simulink model "Final_Tune_of_Bandwidth_PI_Result"  (R2022b)
settings: Solver=FixedStepDiscrete  StartTime=0.0  StopTime=Inf  FixedStep=100e-6  RelTol=1e-3  EnableMultiTasking=on
undefined symbols (not defined in the file): C28x, CPU1, CPU2, CurrentBypassValue, DiscIntNeverNeededParam, Down, GPTRIP1SEL, TZ1, Up
libraries: c2802xlib x20, simulink x16, dspstat3 x10, dspsigops x6, c2837xDlib x5, PID_Lib x5, c280xlib x3, c2000lib x1
(part 1 of 3)
settings Model: ExtModeTrigDuration=8  Creator=user  LastModifiedBy=user
settings SolverCC: AutoInsertRateTranBlk=on
settings OptimizationCC: DefaultParameterBehavior=Inlined  DefaultUnderspecifiedDataType=single  EnhancedBackFolding=on  PassReuseOutputArgsAs=Individual arguments  MaxStackSize=1024  OptimizeBlockOrder=speed  DifferentSizesBufferReuse=on  OptimizationCustomize=off  DenormalBehavior=FlushToZero  EfficientTunableParamExpr=on
settings DebuggingCC: ParameterTunabilityLossMsg=error
settings HardwareCC: ProdBitPerChar=16  ProdBitPerInt=16  ProdBitPerPointer=32  ProdBitPerSizeT=32  ProdBitPerPtrDiffT=32  ProdLargestAtomicInteger=Integer  ProdLargestAtomicFloat=None  ProdWordSize=16  ProdLongLongMode=on  ProdHWDeviceType=Texas Instruments->C2000
settings ModelReferenceCC: ModelReferenceNumInstancesAllowed=Single
settings SFSimCC: MATLABDynamicMemAlloc=off
settings RTWCC: Description=Embedded Coder  SystemTargetFile=ert.tlc  HardwareBoard=TI Delfino F28379D LaunchPad  TLCOptions=-aInlineSetEventsForThisBaseRateFcn=TLC_FALSE -aSuppressMultiTaskScheduler=TLC_FALSE -aRateBasedStepFcn=1  TemplateMakefile=ert_default_tmf  GenerateReport=on  Toolchain=Texas Instruments Code Composer Studio (C2000)  LaunchReport=on
settings CodeAppCC: ForceParamTrailComments=on  IgnoreCustomStorageClasses=off  OperatorAnnotations=on  SimulinkDataObjDesc=on  SFDataObjDesc=on  InsertBlockDesc=on
settings ERTTargetCC: CodeReplacementLibrary=TI C28x  ExtModeTransport=4  ExtModeStaticAlloc=on  ExtModeStaticAllocSize=10000  ExtModeMexFile=ext_xcp  ExtModeIntrfLevel=Level2 - Open  InlinedParameterPlacement=NonHierarchical

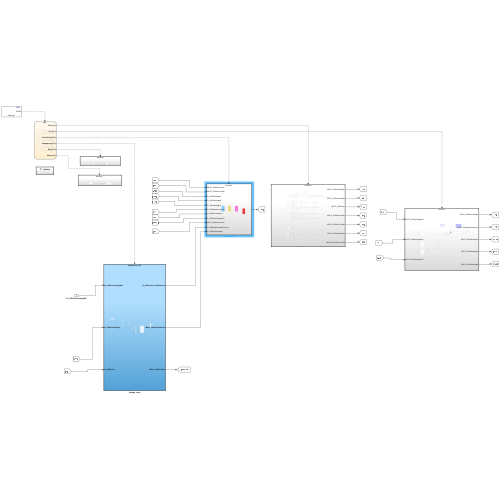
[thumbnail: Simulink's stored preview of the top-level diagram]
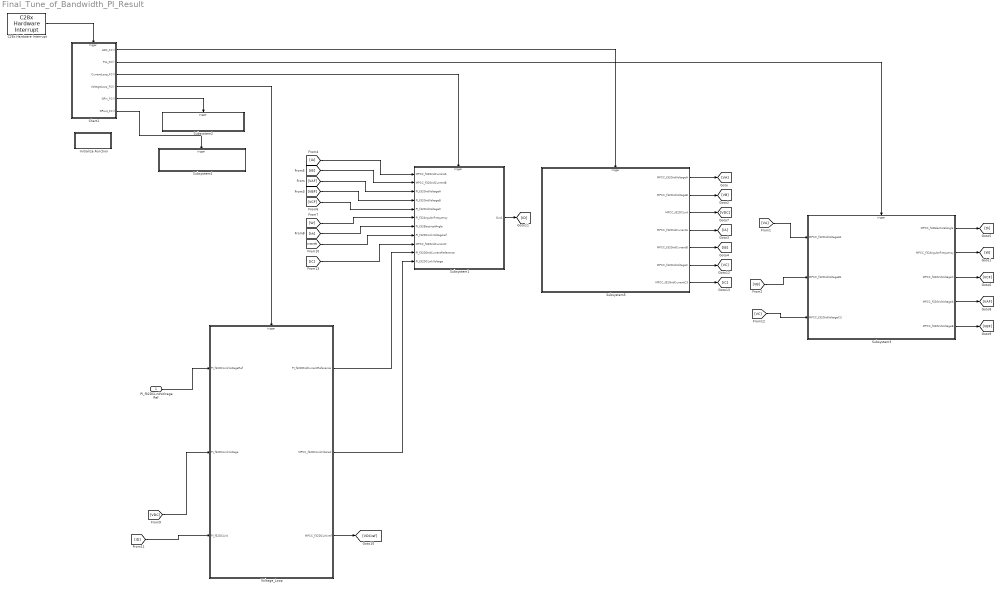
== system Final_Tune_of_Bandwidth_PI_Result ==
  PI_f32DCLinkVoltageRef : Inport
  C28x Hardware Interrupt : c2000lib/Scheduling/C28x Hardware Interrupt  irqnumbers=[1]  pienumbers=[1]  irqpriorities=[1]  irqpreempts=[1]  showinput=off  dspchiptype=C280X
  Chart1 : Stateflow chart  TreatAsAtomicUnit=on
  Initialize Function : Subsystem  TreatAsAtomicUnit=on
  Subsystem1 : Subsystem
  Subsystem2 : Subsystem
  Subsystem3 : Subsystem
  Subsystem4 : Subsystem
  Subsystem5 : Subsystem
  Voltage_Loop : Subsystem
  wires:
  Chart1/5(GPin_FC()) -> Subsystem2/Trigger
  Chart1/3(CurrentLoop_FC()) -> Subsystem1/Trigger
  Chart1/4(VoltageLoop_FC()) -> Voltage_Loop/Trigger
  C28x Hardware Interrupt/1 -> Chart1/Trigger
  Chart1/6(GPout_FC()) -> Subsystem4/Trigger
  Chart1/2(PLL_FC()) -> Subsystem3/Trigger
  Chart1/1(ADC_FC()) -> Subsystem5/Trigger
  Subsystem5/1(MPCC_f32GridVoltageA) -> [VA]
  Subsystem5/2(MPCC_f32GridVoltageB) -> [VB]
  [IA] -> Subsystem1/1(MPCC_f32GridCurrentA)
  [IB] -> Subsystem1/2(MPCC_f32GridCurrentB)
  [W] -> Subsystem1/6(PI_f32AngularFrequency)
  [th] -> Subsystem1/7(PI_f32ElectricalAngle)
  Subsystem5/3(MPCC_f32DCLink) -> [VDC]
  Voltage_Loop/2(MPCC_f32DCLinkFiltered) -> Subsystem1/11(PI_f32DCLinkVoltage)
  [VA] -> Subsystem3/1(MPCC_f32GridVoltageA2)
  [VAF] -> Subsystem1/3(PI_f32GridVoltageA)
  [VCF] -> Subsystem1/5(PI_f32GridVoltageC)
  [VBF] -> Subsystem1/4(PI_f32GridVoltageB)
  Subsystem5/4(MPCC_f32GridCurrentA) -> [IA]
  Subsystem5/5(MPCC_f32GridCurrentB) -> [IB]
  Voltage_Loop/3(MPCC_f32DCLinkref) -> [VDCref]
  [VDCref] -> Subsystem1/8(PI_f32DCLinkVoltageref)
  [VDC] -> Voltage_Loop/2(PI_f32DCLinkVoltage)
  PI_f32DCLinkVoltageRef/1 -> Voltage_Loop/1(PI_f32DCLinkVoltageRef)
  Voltage_Loop/1(PI_f32DGridCurrentReference) -> Subsystem1/10(PI_f32DGridCurrentReference)
  Subsystem1/1(Out1) -> [ID]
  [ID] -> Voltage_Loop/3(PI_f32DCLink)
  [VB] -> Subsystem3/2(MPCC_f32GridVoltageB1)
  Subsystem5/6(MPCC_f32GridVoltageC) -> [VC]
  Subsystem5/7(MPCC_f32GridCurrentC3) -> [IC]
  [VC] -> Subsystem3/3(MPCC_f32GridVoltageC3)
  [IC] -> Subsystem1/9(MPCC_f32GridCurrentC)
  Subsystem3/1(MPCC_f32ElectricalAngle) -> [th]
  Subsystem3/2(MPCC_f32AngularFrequency) -> [W]
  Subsystem3/3(MPCC_f32GridVoltageC) -> [VCF]
  Subsystem3/4(MPCC_f32GridVoltageA) -> [VAF]
  Subsystem3/5(MPCC_f32GridVoltageB) -> [VBF]

== system Final_Tune_of_Bandwidth_PI_Result/Initialize Function ==
  Constant : Constant  Value=boolean(0)
  Digital Output : c2837xDlib/Digital Output  GPIO_Number=GPIO8~GPIO15  GPIO_Bit0=off  GPIO_BIT0_Toggle=off  GPIO_Bit1=off  GPIO_BIT1_Toggle=off  GPIO_Bit2=off  GPIO_BIT2_Toggle=off  GPIO_Bit3=on  GPIO_BIT3_Toggle=off  GPIO_Bit4=off  GPIO_BIT4_Toggle=off  GPIO_Bit5=off  GPIO_BIT5_Toggle=off  GPIO_Bit6=off  GPIO_BIT6_Toggle=off  GPIO_Bit7=off  GPIO_BIT7_Toggle=off
  Event Listener : EventListener  DisableCoverage=on  EventName=reset
  wires:
  Constant/1 -> Digital Output/1

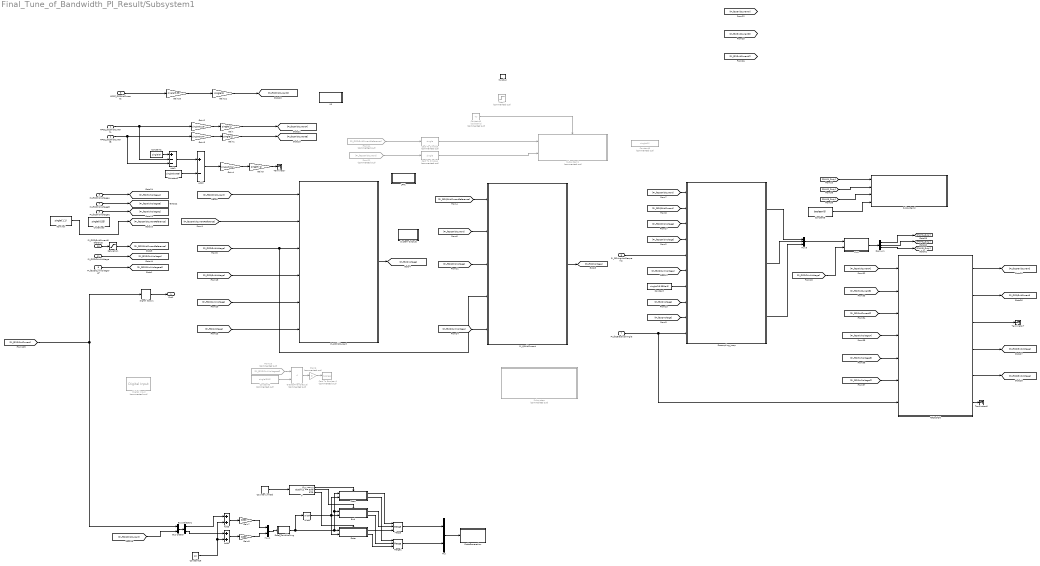
== system Final_Tune_of_Bandwidth_PI_Result/Subsystem1 ==
  MPCC_f32GridCurrentA : Inport
  MPCC_f32GridCurrentB : Inport  Port=2
  PI_f32GridVoltageA : Inport  Port=3
  PI_f32GridVoltageB : Inport  Port=4
  PI_f32GridVoltageC : Inport  Port=5
  PI_f32AngularFrequency : Inport  Port=6
  PI_f32ElectricalAngle : Inport  Port=7
  PI_f32DCLinkVoltageref : Inport  Port=8
  MPCC_f32GridCurrentC : Inport  Port=9
  PI_f32DGridCurrentReference : Inport  Port=10
  PI_f32DCLinkVoltage : Inport  Port=11
  function : TriggerPort  TriggerType=function-call  VariantControl=(inherit)
  ABCtoDQO : Subsystem
  Add1 : Sum  Inputs=+--
  Add2 : Sum  Inputs=+-
  Add3 : Sum
  Add4 : Sum
  Bus Creator : BusCreator  Inputs=2
  Bus Selector1 : BusSelector  OutputSignals=signal1,signal2
  Cast To Boolean1 : DataTypeConversion  Commented=on  OutDataTypeStr=boolean  SaturateOnIntegerOverflow=off  RndMeth=Floor
  Cast To Single3 : DataTypeConversion  Commented=on  OutDataTypeStr=single  SaturateOnIntegerOverflow=off  RndMeth=Floor
  Cast To Single4 : DataTypeConversion  Commented=on  OutDataTypeStr=single  SaturateOnIntegerOverflow=off  RndMeth=Floor
  CodeGeneration : Subsystem  TreatAsAtomicUnit=on
  Constant : Constant  Value=single(18.355e-3)
  Constant1 : Constant  Value=single(0)
  Constant16 : Constant  Value=10  OutDataTypeStr=single
  Constant2 : Constant  Value=single(0.005)
  Constant3 : Constant  Commented=on  Value=boolean(1)
  Constant5 : Constant  Value=boolean(0)
  Constant6 : Constant  Commented=on  Value=single(300)
  Constant9 : Constant  Commented=on  Value=single(0)
  Counter Limited : simulink/Sources/Counter Limited  uplimit=599  tsamp=-1
  Data : Subsystem  TreatAsAtomicUnit=on
  Data_Conditioning : Subsystem
  Decoupling_Loop : Subsystem
  Demux1 : Demux  Outputs=3
  Digital Input : c280xlib/Digital Input  Commented=on  GPIO_Number=GPIO32~GPIO34  GPIO_Bit0=on  GPIO_Bit1=off  GPIO_Bit2=off  GPIO_Bit3=off  GPIO_Bit4=off  GPIO_Bit5=off  GPIO_Bit6=off  GPIO_Bit7=off  sampleTime=-1  dataType=boolean  GPIO_Bit0_Qualification=Sync to SYSCLKOUT  GPIO_Bit1_Qualification=Sync to SYSCLKOUT  GPIO_Bit2_Qualification=Sync to SYSCLKOUT  GPIO_Bit3_Qualification=Sync to SYSCLKOUT  GPIO_Bit4_Qualification=Sync to SYSCLKOUT  GPIO_Bit5_Qualification=Sync to SYSCLKOUT  GPIO_Bit6_Qualification=Sync to SYSCLKOUT  GPIO_Bit7_Qualification=Sync to SYSCLKOUT  Qualification_Period=-1
  End : Subsystem  TreatAsAtomicUnit=on
  From14 : From  Commented=on  GotoTag=PI_f32DGridCurrentReference
  From16 : From  Commented=on  GotoTag=PI_f32DCLinkVoltageref
  From21 : From  Commented=on  GotoTag=PI_f32DGridCurrent
  Gain : Gain  Gain=single(1)
  Gain1 : Gain  Gain=single(1)
  Gain2 : Gain  Gain=single(6.25)
  Gain20 : Gain  Gain=single(5.85)
  Gain21 : Gain  Gain=single(1)
  Gain3 : Gain  Gain=single(5.94)
  Gain4 : Gain  Gain=single(5.94)
  Gain5 : Gain  Gain=single(-1)
  Gain6 : Gain  Commented=on  Gain=0
  Gain7 : Gain  Gain=1000  OutDataTypeStr=single
  Gain8 : Gain  Gain=1000  OutDataTypeStr=single
  GreaterThanOrEqual : RelationalOperator  Commented=on  Operator=<  OutDataTypeStr=boolean  RndMeth=Simplest  InputSameDT=off
  IIR : Subsystem
  If : If  IfExpression=u1 == 0  ElseIfExpressions=u1 == 599
  LPF1 : Subsystem
  Merge : Merge  Inputs=3
  Merge1 : Merge  Inputs=3
  Mux : Mux  Inputs=2
  Mux1 : Mux  Inputs=2
  Mux5 : Mux  Inputs=3
  Nominal : Constant  Value=single(1.1)  VectorParams1D=off  SampleTime=-1
  PI_DGridCurrent : Subsystem
  PI_QGridCurrent : Subsystem
  SVM : Subsystem
  Saturation : Saturate  UpperLimit=7  LowerLimit=-7
  Signal Copy1 : SignalConversion  OverrideOpt=off
  Start : Subsystem  TreatAsAtomicUnit=on
  Step1 : Step  Commented=on  Time=70
  Subsystem : Subsystem  Commented=on
  Subsystem1 : Subsystem  Commented=on
  Subsystem2 : Subsystem
  System Outputs : Subsystem  mask(System Outputs){ShowInLibBrowser=0}
      mask prompts: ShowInLibBrowser "Simulink:masks:CustCodeMaskParam1_MP"
      settings: CopyFcn=cccopyfcn(gcb)  OpenFcn=ccopenfcn('System Outputs Function')
      mask Help: eval('feval(''rtwprivate'',''rtwhelpview'',''rtw_sys_outputs_block'')');
      mask Display: disp('System\nOutputs');
  Terminator : Terminator
  Terminator6 : Terminator
  Terminator7 : Terminator
  Underload : Constant  Value=single(0.55)  VectorParams1D=off  SampleTime=-1
  Width : Width  OutDataTypeMode=All ports same datatype  DataType=uint16
  Out1 : Outport
  wires:
  Add1/1 -> Add2/1
  Gain2/1 -> Gain/1  "Iau"
  Constant2/1 -> Add2/2
  Add2/1 -> Gain4/1
  Gain4/1 -> Gain5/1  "Icu"
  MPCC_f32GridCurrentA/1 -> Gain2/1, Add1/2
  Gain3/1 -> Gain1/1  "Ibu"
  MPCC_f32GridCurrentB/1 -> Add1/3, Gain3/1
  Constant1/1 -> Add1/1
  [PI_f32QGridVoltage] -> Decoupling_Loop/4(PI_f32QGridVoltage)
  [PI_f32QVoltage] -> Decoupling_Loop/9(PI_f32QVoltage)
  [PI_f32QGridCurrentReference] -> PI_QGridCurrent/1(PI_f32QGridCurrentReference)
  [PI_f32QGridCurrent] -> Decoupling_Loop/2(PI_f32QGridCurrent)
  [PI_f32QGridCurrent] -> PI_QGridCurrent/2(PI_f32QGridCurrent)
  [PI_f32DGridVoltage] -> Decoupling_Loop/3(PI_f32DGridVoltage)
  Constant/1 -> Decoupling_Loop/7(PI_f32LGrid)
  [PI_f32DCLinkVoltage] -> Decoupling_Loop/6(PI_f32DCLinkVoltage)
  [PI_f32DGridCurrent] -> Decoupling_Loop/1(PI_f32DGridCurrent)
  PI_QGridCurrent/1(PI_f32QVoltage) -> [PI_f32QVoltage]
  PI_f32AngularFrequency/1 -> Decoupling_Loop/5(PI_f32AngularFrequency)
  PI_DGridCurrent/1(PI_f32DVoltage) -> [PI_f32DVoltage]
  [PI_f32DVoltage] -> Decoupling_Loop/8(PI_f32DVoltage)
  [PI_f32GridCurrentA] -> ABCtoDQO/1(PI_f32GridCurrentA)
  ABCtoDQO/6(PI_f32OGridVoltage) -> Terminator6/1
  [PI_f32GridVoltageB] -> ABCtoDQO/5(PI_f32GridVoltageB)
  ABCtoDQO/1(PI_f32DGridCurrent) -> [PI_f32DGridCurrent]
  [PI_f32GridVoltageC] -> ABCtoDQO/6(PI_f32GridVoltageC)
  ABCtoDQO/5(PI_f32QGridVoltage) -> [PI_f32QGridVoltage]
  [PI_f32GridCurrentB] -> ABCtoDQO/2(PI_f32GridCurrentB)
  [PI_f32GridCurrentC] -> ABCtoDQO/3(PI_f32GridCurrentC)
  ABCtoDQO/3(PI_f32OGridCurrent) -> Terminator7/1
  ABCtoDQO/2(PI_f32QGridCurrent) -> [PI_f32QGridCurrent]
  ABCtoDQO/4(PI_f32DGridVoltage) -> [PI_f32DGridVoltage]
  PI_f32GridVoltageC/1 -> [PI_f32GridVoltageC]
  PI_f32GridVoltageB/1 -> [PI_f32GridVoltageB]
  PI_f32GridVoltageA/1 -> [PI_f32GridVoltageA]
  Gain/1 -> [PI_f32GridCurrentA]
  Gain1/1 -> [PI_f32GridCurrentB]
  Gain5/1 -> Terminator/1
  PI_f32ElectricalAngle/1 -> ABCtoDQO/7(PI_f32ElectricalAngle), Decoupling_Loop/10(PI_f32ElectricalAngle)
  [PI_f32DGridCurrent] -> PI_DGridCurrent/1(PI_f32DGridCurrent)
  PI_f32DCLinkVoltage/1 -> [PI_f32DCLinkVoltage]
  [PI_f32DGridVoltage] -> PI_QGridCurrent/4(PI_f32DGridVoltage), PI_DGridCurrent/3(PI_f32DGridVoltage)
  [PI_f32QGridVoltage] -> PI_QGridCurrent/3(PI_f32QGridVoltage)
  [PI_f32QGridVoltage] -> PI_DGridCurrent/4(PI_f32QGridVoltage)
  [PI_f32GridVoltageA] -> ABCtoDQO/4(PI_f32GridVoltageA)
  [PI_f32DCLinkVoltage] -> PI_DGridCurrent/5(PI_f32DCLinkVoltage)
  [PI_f32QVoltage] -> PI_DGridCurrent/6(PI_f32QVoltage)
  [PI_f32DCLinkVoltage] -> PI_QGridCurrent/5(PI_f32DCLinkVoltage)
  PI_f32DCLinkVoltageref/1 -> [PI_f32DCLinkVoltageref]
  Saturation/1 -> [PI_f32DGridCurrentReference]
  PI_f32DGridCurrentReference/1 -> Saturation/1
  From16/1 -> GreaterThanOrEqual/1
  Constant6/1 -> GreaterThanOrEqual/2
  GreaterThanOrEqual/1 -> Gain6/1
  Cast To Single4/1 -> Subsystem1/2(In2)
  Cast To Single3/1 -> Subsystem1/1(In1)
  From21/1 -> Cast To Single4/1
  From14/1 -> Cast To Single3/1
  Signal Copy1/1 -> Out1/1
  Constant3/1 -> Subsystem1/Enable
  MPCC_f32GridCurrentC/1 -> Gain20/1
  Gain21/1 -> [PI_f32GridCurrentC]  "Iau"
  Gain20/1 -> Gain21/1  "Iau"
  Gain6/1 -> Cast To Boolean1/1
  Demux1/2 -> [PWM2_Duty]
  SVM/1(Dabc) -> Demux1/1
  Demux1/3 -> [PWM3_Duty]
  Demux1/1 -> [PWM1_Duty]
  Decoupling_Loop/2(PI_f32MBVoltageRef) -> Mux5/2
  Decoupling_Loop/1(PI_f32MAVoltageRef) -> Mux5/1
  Decoupling_Loop/3(PI_f32MCVoltageRef) -> Mux5/3
  Mux5/1 -> SVM/1(Vabc)
  [PI_f32DCLinkVoltage] -> SVM/2(Vdc)
  [PWM1_Duty] -> Subsystem2/1(PWM1)
  [PWM2_Duty] -> Subsystem2/2(PWM2)
  [PWM3_Duty] -> Subsystem2/3(PWM3)
  Constant5/1 -> Subsystem2/4(Trip)
  [PI_f32DGridCurrent] -> Signal Copy1/1, Bus Creator/1
  [PI_f32DGridCurrentReference] -> PI_DGridCurrent/2(PI_f32DGridCurrentReference)
  Start/2(Iteration) -> Merge1/1
  Gain8/1 -> Mux1/2
  Data/2(Iteration) -> Merge1/3
  Bus Selector1/1 -> Add3/1  "<signal1>"
  Counter Limited/1 -> If/1
  If/3 -> Data/Action
  End/1(Data_out) -> Merge/2
  If/1 -> Start/Action
  If/2 -> End/Action
  Width/1 -> Data/2(Data_width), Start/2(Data_width), End/2(Data_width)
  Data_Conditioning/1(Out1) -> Width/1, Start/1(Data), End/1(Data), Data/1(Data)
  Merge/1 -> Mux/1  "SCI_Tx_Data"
  End/2(Iteration) -> Merge1/2
  Merge1/1 -> Mux/2  "SCI_Tx_Iteration"
  Start/1(Data_out) -> Merge/1
  Add3/1 -> Gain7/1
  Bus Creator/1 -> Bus Selector1/1
  Gain7/1 -> Mux1/1
  Mux/1 -> CodeGeneration/1(Input)
  Constant16/1 -> Add3/2, Add4/2
  Bus Selector1/2 -> Add4/1  "<signal2>"
  Data/1(Data_out) -> Merge/3
  Mux1/1 -> Data_Conditioning/1(In1)
  [PI_f32QGridCurrent] -> Bus Creator/2
  Add4/1 -> Gain8/1
  Nominal/1 -> [PI_f32QGridCurrentReference]

== system Final_Tune_of_Bandwidth_PI_Result/Subsystem2 ==
  function : TriggerPort  TriggerType=function-call  VariantControl=(inherit)
  Constant : Constant  Value=boolean(1)
  Digital Output : c2837xDlib/Digital Output  GPIO_Number=GPIO8~GPIO15  GPIO_Bit0=off  GPIO_BIT0_Toggle=off  GPIO_Bit1=off  GPIO_BIT1_Toggle=off  GPIO_Bit2=off  GPIO_BIT2_Toggle=off  GPIO_Bit3=off  GPIO_BIT3_Toggle=off  GPIO_Bit4=off  GPIO_BIT4_Toggle=off  GPIO_Bit5=off  GPIO_BIT5_Toggle=off  GPIO_Bit6=on  GPIO_BIT6_Toggle=off  GPIO_Bit7=off  GPIO_BIT7_Toggle=off
  wires:
  Constant/1 -> Digital Output/1

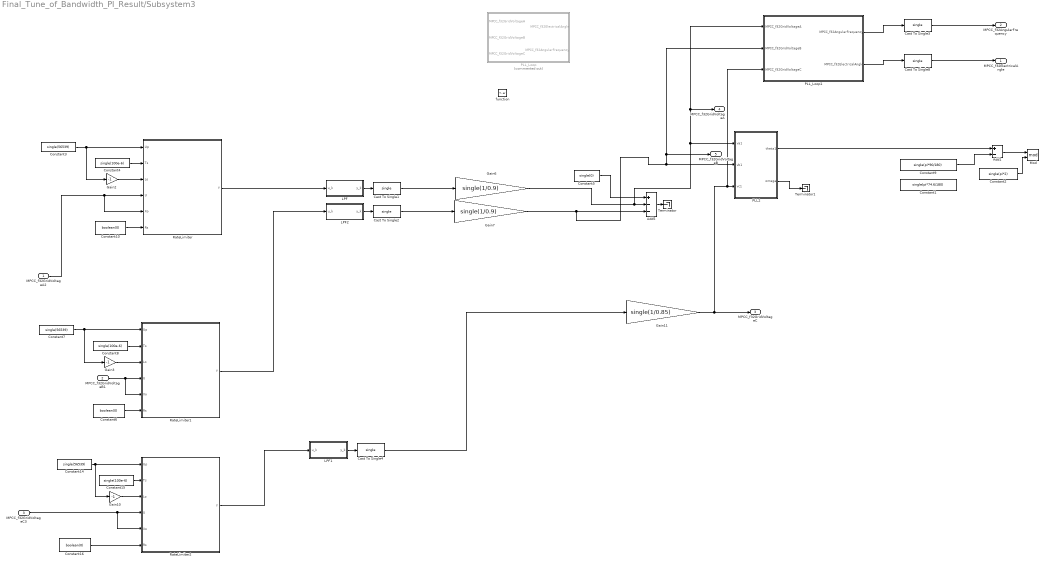
== system Final_Tune_of_Bandwidth_PI_Result/Subsystem3 ==
  MPCC_f32GridVoltageA2 : Inport
  MPCC_f32GridVoltageB1 : Inport  Port=2
  MPCC_f32GridVoltageC3 : Inport  Port=3
  function : TriggerPort  TriggerType=function-call  VariantControl=(inherit)
  Add1 : Sum  Inputs=+-
  Add5 : Sum  Inputs=+--
  Cast To Single{1..4,8} (5 alike) : DataTypeConversion  OutDataTypeStr=single  SaturateOnIntegerOverflow=off  RndMeth=Floor
  Constant1 : Constant  Value=single(pi*74.6/180)
  Constant10 : Constant  Value=boolean(0)
  Constant14 : Constant  Value=single(56539)
  Constant15 : Constant  Value=single(100e-6)
  Constant16 : Constant  Value=boolean(0)
  Constant2 : Constant  Value=single(pi*2)
  Constant3 : Constant  Value=single(56539)
  Constant4 : Constant  Value=single(100e-6)
  Constant5 : Constant  Value=single(0)
  Constant6 : Constant  Value=boolean(0)
  Constant7 : Constant  Value=single(56539)
  Constant8 : Constant  Value=single(100e-6)
  Constant9 : Constant  Value=single(pi*90/180)
  Gain10 : Gain  Gain=-1
  Gain11 : Gain  Gain=single(1/0.85)
  Gain2 : Gain  Gain=-1
  Gain3 : Gain  Gain=-1
  Gain6 : Gain  Gain=single(1/0.9)
  Gain7 : Gain  Gain=single(1/0.9)
  LPF : Subsystem
  LPF1 : Subsystem
  LPF2 : Subsystem
  Mod : Math  Operator=mod
  PLL2 : Subsystem
  PLL_Loop : Subsystem  Commented=on  TreatAsAtomicUnit=on
  PLL_Loop1 : Subsystem
  RateLimiter : Subsystem
  RateLimiter1 : Subsystem
  RateLimiter2 : Subsystem
  Terminator : Terminator
  Terminator1 : Terminator
  MPCC_f32ElectricalAngle : Outport
  MPCC_f32AngularFrequency : Outport  Port=2
  MPCC_f32GridVoltageC : Outport  Port=3
  MPCC_f32GridVoltageA : Outport  Port=4
  MPCC_f32GridVoltageB : Outport  Port=5
  wires:
  Cast To Single1/1 -> Gain6/1
  Constant5/1 -> Add5/1
  Cast To Single2/1 -> Gain7/1
  Constant2/1 -> Mod/2
  PLL2/1(theta1) -> Add1/1
  Add1/1 -> Mod/1
  LPF/1(y_k) -> Cast To Single1/1
  LPF2/1(y_k) -> Cast To Single2/1
  Gain6/1 -> PLL_Loop1/1(MPCC_f32GridVoltageA), MPCC_f32GridVoltageA/1, PLL2/1(va1), Add5/2
  Gain7/1 -> MPCC_f32GridVoltageB/1, PLL_Loop1/2(MPCC_f32GridVoltageB), PLL2/2(vb1), Add5/3
  Gain2/1 -> RateLimiter/3(Lo)
  Constant10/1 -> RateLimiter/6(Rs)
  Constant3/1 -> Gain2/1, RateLimiter/1(Up)
  Constant4/1 -> RateLimiter/2(Ts)
  MPCC_f32GridVoltageA2/1 -> RateLimiter/5(Xo), RateLimiter/4(U)
  RateLimiter/1(Y) -> LPF/1(u_k)
  Constant7/1 -> Gain3/1, RateLimiter1/1(Up)
  Constant6/1 -> RateLimiter1/6(Rs)
  Constant8/1 -> RateLimiter1/2(Ts)
  Gain3/1 -> RateLimiter1/3(Lo)
  MPCC_f32GridVoltageB1/1 -> RateLimiter1/5(Xo), RateLimiter1/4(U)
  RateLimiter1/1(Y) -> LPF2/1(u_k)
  MPCC_f32GridVoltageC3/1 -> RateLimiter2/5(Xo), RateLimiter2/4(U)
  Cast To Single4/1 -> Gain11/1
  LPF1/1(y_k) -> Cast To Single4/1
  Constant14/1 -> Gain10/1, RateLimiter2/1(Up)
  Constant15/1 -> RateLimiter2/2(Ts)
  Constant16/1 -> RateLimiter2/6(Rs)
  Gain10/1 -> RateLimiter2/3(Lo)
  RateLimiter2/1(Y) -> LPF1/1(u_k)
  Add5/1 -> Terminator/1
  Gain11/1 -> PLL2/3(vc1), PLL_Loop1/3(MPCC_f32GridVoltageC), MPCC_f32GridVoltageC/1
  Constant9/1 -> Add1/2
  Cast To Single8/1 -> MPCC_f32ElectricalAngle/1
  Cast To Single3/1 -> MPCC_f32AngularFrequency/1
  PLL_Loop1/2(MPCC_f32ElectricalAngle) -> Cast To Single8/1
  PLL_Loop1/1(MPCC_f32AngularFrequency) -> Cast To Single3/1
  PLL2/2(omega) -> Terminator1/1

== system Final_Tune_of_Bandwidth_PI_Result/Subsystem4 ==
  function : TriggerPort  TriggerType=function-call  VariantControl=(inherit)
  Constant : Constant  Value=boolean(0)
  Digital Output : c2837xDlib/Digital Output  GPIO_Number=GPIO8~GPIO15  GPIO_Bit0=off  GPIO_BIT0_Toggle=off  GPIO_Bit1=off  GPIO_BIT1_Toggle=off  GPIO_Bit2=off  GPIO_BIT2_Toggle=off  GPIO_Bit3=off  GPIO_BIT3_Toggle=off  GPIO_Bit4=off  GPIO_BIT4_Toggle=off  GPIO_Bit5=off  GPIO_BIT5_Toggle=off  GPIO_Bit6=on  GPIO_BIT6_Toggle=off  GPIO_Bit7=off  GPIO_BIT7_Toggle=off
  wires:
  Constant/1 -> Digital Output/1

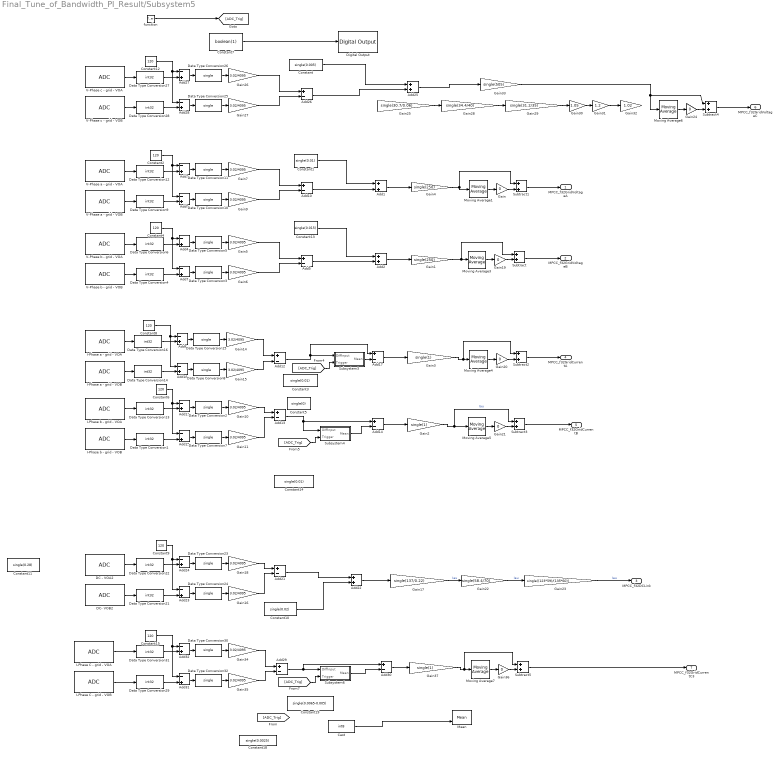
== system Final_Tune_of_Bandwidth_PI_Result/Subsystem5 ==
  function : TriggerPort  TriggerType=function-call  VariantControl=(inherit)  ShowOutputPort=on  OutputDataType=int8
  Add{1..2,22,25} (4 alike) : Sum  AccumDataTypeStr=single  OutDataTypeStr=single
  Add{5,10,12..14,17,21,26,29..30} (10 alike) : Sum  Inputs=+-  AccumDataTypeStr=single  OutDataTypeStr=single
  Add{3..4,6..7,9,11,15,18,23..24,27..28,31..32} (14 alike) : Sum  Inputs=-+  AccumDataTypeStr=single  OutDataTypeStr=single
  Cast : DataTypeConversion  OutDataTypeStr=int8  SaturateOnIntegerOverflow=off  RndMeth=Floor
  Constant : Constant  Value=single(0.005)
  Constant1 : Constant  Value=single(0.01)
  Constant10 : Constant  Value=single(0.02)
  Constant11 : Constant  Value=single(0.28)
  Constant{2,4,6,8..9,12,15} (7 alike) : Constant  Value=120  OutDataTypeStr=single
  Constant13 : Constant  Value=single(0.015)
  Constant14 : Constant  Value=single(0.01)
  Constant18 : Constant  Value=single(0.0025)
  Constant19 : Constant  Value=single(0.0065-0.005)
  Constant3 : Constant  Value=single(0.01)
  Constant5 : Constant  Value=single(0)
  Constant7 : Constant  Value=boolean(1)
  DC - VOA2 : c2802xlib/ADC  blkParamProc=C2000_Type4  ADCModule=C  samplingMode=Single sample mode  ADCResolution=12-bit (Single-ended input)  useSOC1=SOC0  useSOC2=SOC0_SOC1  SOCAcquisitionWindow=22  SOCTriggerSource=ePWM1_ADCSOCA  SOCInterruptTrigger=No ADCINT  Ts=-1  dType=uint16  postInterrupt=off  interruptSel=ADCINT1  ADCINTContinuous=on  endma=off  chdma=1  conv1=ADCINA0  conv2=ADCINA0 and ADCINB0  conv1_Type4=ADCIN5  conv2_Type4=ADCIN0 and ADCIN1
  DC- VOB2 : c2802xlib/ADC  blkParamProc=C2000_Type4  ADCModule=B  samplingMode=Single sample mode  ADCResolution=12-bit (Single-ended input)  useSOC1=SOC3  useSOC2=SOC0_SOC1  SOCAcquisitionWindow=22  SOCTriggerSource=ePWM1_ADCSOCA  SOCInterruptTrigger=No ADCINT  Ts=-1  dType=uint16  postInterrupt=off  interruptSel=ADCINT2  ADCINTContinuous=on  endma=off  chdma=1  conv1=ADCINA0  conv2=ADCINA0 and ADCINB0  conv1_Type4=ADCIN5  conv2_Type4=ADCIN2 and ADCIN3
  Data Type Conversion{1,4,6,9,12..14,16,21..22,27..29,31} (14 alike) : DataTypeConversion  OutDataTypeStr=int32  ConvertRealWorld=Stored Integer (SI)  SaturateOnIntegerOverflow=off  RndMeth=Floor
  Data Type Conversion{2..3,5,7..8,10..11,15,23..26,30,32} (14 alike) : DataTypeConversion  OutDataTypeStr=single  SaturateOnIntegerOverflow=off  RndMeth=Floor
  Digital Output : c2837xDlib/Digital Output  GPIO_Number=GPIO32~GPIO39  GPIO_Bit0=on  GPIO_BIT0_Toggle=on  GPIO_Bit1=off  GPIO_BIT1_Toggle=off  GPIO_Bit2=off  GPIO_BIT2_Toggle=off  GPIO_Bit3=off  GPIO_BIT3_Toggle=off  GPIO_Bit4=off  GPIO_BIT4_Toggle=off  GPIO_Bit5=off  GPIO_BIT5_Toggle=off  GPIO_Bit6=off  GPIO_BIT6_Toggle=off  GPIO_Bit7=off  GPIO_BIT7_Toggle=off
  Gain{,19..21,24,36} (6 alike) : Gain  Gain=0
  Gain1 : Gain  Gain=single(250)
  Gain{5..7,9..11,14..16,18,26..27,34..35} (14 alike) : Gain  Gain=3.02/4095  ParamDataTypeStr=single  OutDataTypeStr=single
  Gain17 : Gain  Gain=single(137/0.22)
  Gain2 : Gain  Gain=single(1)
  Gain22 : Gain  Gain=single(58.4/70)
  Gain23 : Gain  Gain=single((123*59)/(135*60))
  Gain25 : Gain  Gain=single(30.7/0.06)
  Gain28 : Gain  Gain=single(34.4/40)
  Gain29 : Gain  Gain=single(31.2/35)
  Gain3 : Gain  Gain=single(1)
  Gain30 : Gain  Gain=1.05
  Gain31 : Gain  Gain=1.2
  Gain32 : Gain  Gain=1.02
  Gain33 : Gain  Gain=single(505)
  Gain37 : Gain  Gain=single(1)
  Gain4 : Gain  Gain=single(250)
  I-Phase C - grid - VOA : c2802xlib/ADC  blkParamProc=C2000_Type4  ADCModule=A  samplingMode=Single sample mode  ADCResolution=12-bit (Single-ended input)  useSOC1=SOC15  useSOC2=SOC0_SOC1  SOCAcquisitionWindow=22  SOCTriggerSource=ePWM1_ADCSOCA  SOCInterruptTrigger=No ADCINT  Ts=-1  dType=uint16  postInterrupt=off  interruptSel=ADCINT1  ADCINTContinuous=on  endma=off  chdma=1  conv1=ADCINA0  conv2=ADCINA0 and ADCINB0  conv1_Type4=ADCIN15  conv2_Type4=ADCIN0 and ADCIN1
  I-Phase C - grid - VOB : c2802xlib/ADC  blkParamProc=C2000_Type4  ADCModule=A  samplingMode=Single sample mode  ADCResolution=12-bit (Single-ended input)  useSOC1=SOC10  useSOC2=SOC0_SOC1  SOCAcquisitionWindow=22  SOCTriggerSource=ePWM1_ADCSOCA  SOCInterruptTrigger=No ADCINT  Ts=-1  dType=uint16  postInterrupt=off  interruptSel=ADCINT2  ADCINTContinuous=on  endma=off  chdma=1  conv1=ADCINA0  conv2=ADCINA0 and ADCINB0  conv1_Type4=ADCIN14  conv2_Type4=ADCIN2 and ADCIN3
  I-Phase a - grid - VOA : c2802xlib/ADC  blkParamProc=C2000_Type4  ADCModule=A  samplingMode=Single sample mode  ADCResolution=12-bit (Single-ended input)  useSOC1=SOC0  useSOC2=SOC0_SOC1  SOCAcquisitionWindow=22  SOCTriggerSource=ePWM1_ADCSOCA  SOCInterruptTrigger=No ADCINT  Ts=-1  dType=uint16  postInterrupt=on  interruptSel=ADCINT1  ADCINTContinuous=on  endma=off  chdma=1  conv1=ADCINA0  conv2=ADCINA0 and ADCINB0  conv1_Type4=ADCIN4  conv2_Type4=ADCIN0 and ADCIN1
  I-Phase a - grid - VOB : c2802xlib/ADC  blkParamProc=C2000_Type4  ADCModule=B  samplingMode=Single sample mode  ADCResolution=12-bit (Single-ended input)  useSOC1=SOC1  useSOC2=SOC0_SOC1  SOCAcquisitionWindow=22  SOCTriggerSource=ePWM1_ADCSOCA  SOCInterruptTrigger=No ADCINT  Ts=-1  dType=uint16  postInterrupt=off  interruptSel=ADCINT2  ADCINTContinuous=on  endma=off  chdma=1  conv1=ADCINA0  conv2=ADCINA0 and ADCINB0  conv1_Type4=ADCIN4  conv2_Type4=ADCIN2 and ADCIN3
  I-Phase b - grid - VOA : c2802xlib/ADC  blkParamProc=C2000_Type4  ADCModule=C  samplingMode=Single sample mode  ADCResolution=12-bit (Single-ended input)  useSOC1=SOC12  useSOC2=SOC0_SOC1  SOCAcquisitionWindow=22  SOCTriggerSource=ePWM1_ADCSOCA  SOCInterruptTrigger=No ADCINT  Ts=-1  dType=uint16  postInterrupt=off  interruptSel=ADCINT1  ADCINTContinuous=on  endma=off  chdma=1  conv1=ADCINA0  conv2=ADCINA0 and ADCINB0  conv1_Type4=ADCIN4  conv2_Type4=ADCIN0 and ADCIN1
  I-Phase b - grid - VOB : c2802xlib/ADC  blkParamProc=C2000_Type4  ADCModule=A  samplingMode=Single sample mode  ADCResolution=12-bit (Single-ended input)  useSOC1=SOC3  useSOC2=SOC0_SOC1  SOCAcquisitionWindow=22  SOCTriggerSource=ePWM1_ADCSOCA  SOCInterruptTrigger=No ADCINT  Ts=-1  dType=uint16  postInterrupt=off  interruptSel=ADCINT2  ADCINTContinuous=on  endma=off  chdma=1  conv1=ADCINA0  conv2=ADCINA0 and ADCINB0  conv1_Type4=ADCIN5  conv2_Type4=ADCIN2 and ADCIN3
  Mean : dspstat3/Mean  run=on  InputProcessing=Columns as channels (frame based)  reset_popup=Rising edge  directionMode=Each column  dimension=1  roiEnable=off  roiType=Rectangles  roiPortion=Entire ROI  roiOutput=Individual statistics for each ROI  roiFlag=off  roundingMode=Floor  overflowMode=off  outputDataTypeStr=Inherit: Same as accumulator  outputMin=[]  outputMax=[]  outputLastDataTypeStr=Inherit: Same as accumulator
  Moving Average{1,3..7} (6 alike) : dspstat3/Moving Average  Method=Exponential weighting  ForgettingFactorPort=off  SpecifyWindowLength=on  WindowLength=4  OverlapLength=3  AllowArbitraryInputLength=off  ForgettingFactor=0.99  SimulateUsing=Code generation
  Subsystem3 : Subsystem
  Subsystem4 : Subsystem
  Subsystem6 : Subsystem
  Subtract{,1..5} (6 alike) : Sum
  V-Phase a - grid - VOA : c2802xlib/ADC  blkParamProc=C2000_Type4  ADCModule=C  samplingMode=Single sample mode  ADCResolution=12-bit (Single-ended input)  useSOC1=SOC4  useSOC2=SOC0_SOC1  SOCAcquisitionWindow=22  SOCTriggerSource=ePWM1_ADCSOCA  SOCInterruptTrigger=No ADCINT  Ts=-1  dType=uint16  postInterrupt=off  interruptSel=ADCINT1  ADCINTContinuous=on  endma=off  chdma=1  conv1=ADCINA0  conv2=ADCINA0 and ADCINB0  conv1_Type4=ADCIN3  conv2_Type4=ADCIN0 and ADCIN1
  V-Phase a - grid - VOB : c2802xlib/ADC  blkParamProc=C2000_Type4  ADCModule=B  samplingMode=Single sample mode  ADCResolution=12-bit (Single-ended input)  useSOC1=SOC5  useSOC2=SOC0_SOC1  SOCAcquisitionWindow=22  SOCTriggerSource=ePWM1_ADCSOCA  SOCInterruptTrigger=No ADCINT  Ts=-1  dType=uint16  postInterrupt=off  interruptSel=ADCINT2  ADCINTContinuous=on  endma=off  chdma=1  conv1=ADCINA0  conv2=ADCINA0 and ADCINB0  conv1_Type4=ADCIN3  conv2_Type4=ADCIN2 and ADCIN3
  V-Phase b - grid - VOA : c2802xlib/ADC  blkParamProc=C2000_Type4  ADCModule=A  samplingMode=Single sample mode  ADCResolution=12-bit (Single-ended input)  useSOC1=SOC6  useSOC2=SOC0_SOC1  SOCAcquisitionWindow=22  SOCTriggerSource=ePWM1_ADCSOCA  SOCInterruptTrigger=No ADCINT  Ts=-1  dType=uint16  postInterrupt=off  interruptSel=ADCINT1  ADCINTContinuous=on  endma=off  chdma=1  conv1=ADCINA0  conv2=ADCINA0 and ADCINB0  conv1_Type4=ADCIN3  conv2_Type4=ADCIN0 and ADCIN1
  V-Phase b - grid - VOB : c2802xlib/ADC  blkParamProc=C2000_Type4  ADCModule=C  samplingMode=Single sample mode  ADCResolution=12-bit (Single-ended input)  useSOC1=SOC7  useSOC2=SOC0_SOC1  SOCAcquisitionWindow=22  SOCTriggerSource=ePWM1_ADCSOCA  SOCInterruptTrigger=No ADCINT  Ts=-1  dType=uint16  postInterrupt=off  interruptSel=ADCINT2  ADCINTContinuous=on  endma=off  chdma=1  conv1=ADCINA0  conv2=ADCINA0 and ADCINB0  conv1_Type4=ADCIN2  conv2_Type4=ADCIN2 and ADCIN3
  V-Phase c - grid - VOA : c2802xlib/ADC  blkParamProc=C2000_Type4  ADCModule=B  samplingMode=Single sample mode  ADCResolution=12-bit (Single-ended input)  useSOC1=SOC0  useSOC2=SOC0_SOC1  SOCAcquisitionWindow=22  SOCTriggerSource=ePWM1_ADCSOCA  SOCInterruptTrigger=No ADCINT  Ts=-1  dType=uint16  postInterrupt=off  interruptSel=ADCINT1  ADCINTContinuous=on  endma=off  chdma=1  conv1=ADCINA0  conv2=ADCINA0 and ADCINB0  conv1_Type4=ADCIN2  conv2_Type4=ADCIN0 and ADCIN1
  V-Phase c - grid - VOB : c2802xlib/ADC  blkParamProc=C2000_Type4  ADCModule=A  samplingMode=Single sample mode  ADCResolution=12-bit (Single-ended input)  useSOC1=SOC1  useSOC2=SOC0_SOC1  SOCAcquisitionWindow=22  SOCTriggerSource=ePWM1_ADCSOCA  SOCInterruptTrigger=No ADCINT  Ts=-1  dType=uint16  postInterrupt=off  interruptSel=ADCINT2  ADCINTContinuous=on  endma=off  chdma=1  conv1=ADCINA0  conv2=ADCINA0 and ADCINB0  conv1_Type4=ADCIN2  conv2_Type4=ADCIN2 and ADCIN3
  MPCC_f32GridVoltageA : Outport
  MPCC_f32GridVoltageB : Outport  Port=2
  MPCC_f32DCLink : Outport  Port=3
  MPCC_f32GridCurrentA : Outport  Port=4
  MPCC_f32GridCurrentB : Outport  Port=5
  MPCC_f32GridVoltageC : Outport  Port=6
  MPCC_f32GridCurrentC3 : Outport  Port=7
  wires:
  Gain5/1 -> Add5/1
  Data Type Conversion5/1 -> Gain5/1
  Gain1/1 -> Subtract/1, Moving Average3/1
  Add9/1 -> Data Type Conversion10/1
  V-Phase a - grid - VOB/1 -> Data Type Conversion9/1
  Data Type Conversion9/1 -> Add9/2
  Gain7/1 -> Add10/1
  Data Type Conversion10/1 -> Gain9/1
  Data Type Conversion12/1 -> Add3/2
  Add7/1 -> Data Type Conversion3/1
  Data Type Conversion4/1 -> Add7/2
  Data Type Conversion6/1 -> Add4/2
  Gain9/1 -> Add10/2
  V-Phase b - grid - VOB/1 -> Data Type Conversion4/1
  V-Phase b - grid - VOA/1 -> Data Type Conversion6/1
  Add4/1 -> Data Type Conversion5/1
  Add3/1 -> Data Type Conversion11/1
  Data Type Conversion3/1 -> Gain6/1
  Gain6/1 -> Add5/2
  Constant4/1 -> Add7/1, Add4/1
  V-Phase a - grid - VOA/1 -> Data Type Conversion12/1
  Constant2/1 -> Add9/1, Add3/1
  Data Type Conversion11/1 -> Gain7/1
  Add1/1 -> Gain4/1
  Add2/1 -> Gain1/1
  I-Phase b - grid - VOA/1 -> Data Type Conversion13/1
  Data Type Conversion15/1 -> Gain14/1
  Data Type Conversion8/1 -> Gain15/1
  Data Type Conversion14/1 -> Add18/2
  Gain15/1 -> Add12/2
  Data Type Conversion13/1 -> Add11/2
  Data Type Conversion16/1 -> Add6/2
  Gain14/1 -> Add12/1
  Add6/1 -> Data Type Conversion15/1
  Gain10/1 -> Add13/1
  Add18/1 -> Data Type Conversion8/1
  I-Phase a - grid - VOA/1 -> Data Type Conversion16/1
  Gain2/1 -> Subtract3/1, Moving Average5/1  "Iau"
  Data Type Conversion2/1 -> Gain10/1
  Constant6/1 -> Add15/1, Add11/1
  I-Phase b - grid - VOB/1 -> Data Type Conversion1/1
  Data Type Conversion1/1 -> Add15/2
  Gain11/1 -> Add13/2
  Add17/1 -> Gain3/1
  Add11/1 -> Data Type Conversion2/1
  Constant8/1 -> Add18/1, Add6/1
  I-Phase a - grid - VOB/1 -> Data Type Conversion14/1
  Data Type Conversion7/1 -> Gain11/1
  Add15/1 -> Data Type Conversion7/1
  Subtract/1 -> MPCC_f32GridVoltageB/1
  Moving Average3/1 -> Gain19/1
  Moving Average1/1 -> Gain/1
  Gain4/1 -> Subtract1/1, Moving Average1/1
  Subtract1/1 -> MPCC_f32GridVoltageA/1
  Moving Average4/1 -> Gain20/1
  Gain3/1 -> Subtract2/1, Moving Average4/1
  Moving Average5/1 -> Gain21/1
  Data Type Conversion22/1 -> Add24/2
  DC- VOB2/1 -> Data Type Conversion21/1
  Data Type Conversion21/1 -> Add23/2
  Data Type Conversion23/1 -> Gain18/1
  DC - VOA2/1 -> Data Type Conversion22/1
  Add24/1 -> Data Type Conversion23/1
  Constant9/1 -> Add23/1, Add24/1
  Gain16/1 -> Add21/2
  Add23/1 -> Data Type Conversion24/1
  Data Type Conversion24/1 -> Gain16/1
  Gain18/1 -> Add21/1
  Gain/1 -> Subtract1/2
  Gain19/1 -> Subtract/2
  Gain20/1 -> Subtract2/2
  Gain21/1 -> Subtract3/2
  Gain17/1 -> Gain22/1  "Iau"
  Subtract2/1 -> MPCC_f32GridCurrentA/1
  Subtract3/1 -> MPCC_f32GridCurrentB/1
  Gain22/1 -> Gain23/1  "Iau"
  V-Phase c - grid - VOB/1 -> Data Type Conversion28/1
  Gain26/1 -> Add26/1
  Data Type Conversion25/1 -> Gain27/1
  V-Phase c - grid - VOA/1 -> Data Type Conversion27/1
  Subtract4/1 -> MPCC_f32GridVoltageC/1
  Data Type Conversion26/1 -> Gain26/1
  Data Type Conversion27/1 -> Add27/2
  Moving Average6/1 -> Gain24/1
  Data Type Conversion28/1 -> Add28/2
  Gain27/1 -> Add26/2
  Add28/1 -> Data Type Conversion25/1
  Constant12/1 -> Add28/1, Add27/1
  Add27/1 -> Data Type Conversion26/1
  Gain25/1 -> Gain28/1
  Gain24/1 -> Subtract4/2
  Gain28/1 -> Gain29/1
  Gain29/1 -> Gain30/1
  Gain30/1 -> Gain31/1
  Gain31/1 -> Gain32/1
  Gain33/1 -> Subtract4/1, Moving Average6/1
  Add31/1 -> Data Type Conversion32/1
  Data Type Conversion32/1 -> Gain35/1
  Data Type Conversion31/1 -> Add32/2
  Gain34/1 -> Add29/1
  Constant15/1 -> Add31/1, Add32/1
  Gain35/1 -> Add29/2
  Subtract5/1 -> MPCC_f32GridCurrentC3/1
  Gain36/1 -> Subtract5/2
  Data Type Conversion30/1 -> Gain34/1
  Data Type Conversion29/1 -> Add31/2
  I-Phase C - grid - VOB/1 -> Data Type Conversion29/1
  I-Phase C - grid - VOA/1 -> Data Type Conversion31/1
  Gain37/1 -> Subtract5/1, Moving Average7/1
  Add32/1 -> Data Type Conversion30/1
  Add30/1 -> Gain37/1
  Moving Average7/1 -> Gain36/1
  Add22/1 -> Gain17/1
  Constant7/1 -> Digital Output/1
  Add14/1 -> Gain2/1
  function/1 -> [ADC_Trig]
  Cast/1 -> Mean/2
  Add25/1 -> Gain33/1
  [ADC_Trig] -> Subsystem3/2(Trigger)
  Add12/1 -> Add17/1, Subsystem3/1(DiffInput)
  Subsystem3/1(Mean) -> Add17/2
  [ADC_Trig] -> Subsystem4/2(Trigger)
  Add13/1 -> Add14/1, Subsystem4/1(DiffInput)
  Subsystem4/1(Mean) -> Add14/2
  [ADC_Trig] -> Subsystem6/2(Trigger)
  Add29/1 -> Add30/1, Subsystem6/1(DiffInput)
  Subsystem6/1(Mean) -> Add30/2
  Constant/1 -> Add25/1
  Add26/1 -> Add25/2
  Constant1/1 -> Add1/1
  Add10/1 -> Add1/2
  Constant13/1 -> Add2/1
  Add5/1 -> Add2/2
  Gain23/1 -> MPCC_f32DCLink/1  "Iau"
  Add21/1 -> Add22/1
  Constant10/1 -> Add22/2

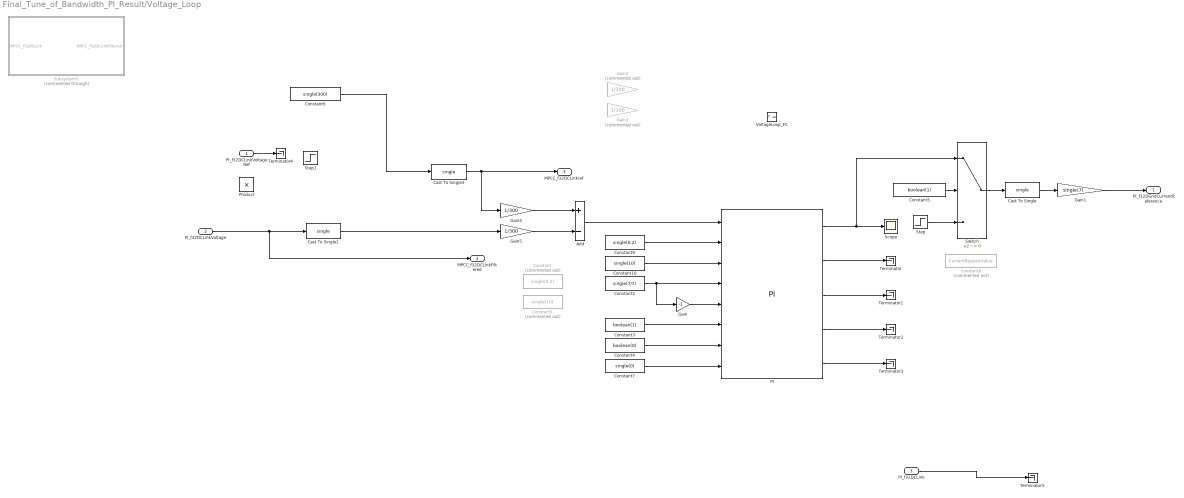
== system Final_Tune_of_Bandwidth_PI_Result/Voltage_Loop ==
  PI_f32DCLinkVoltageRef : Inport
  PI_f32DCLinkVoltage : Inport  Port=2
  PI_f32DCLink : Inport  Port=3
  VoltageLoop_FC : TriggerPort  TriggerType=function-call  VariantControl=(inherit)  SampleTime=-1
      settings: AttributesFormatString=|
      | %<StatesWhenEnabling>
      | %<SampleTime>
  Add : Sum  Inputs=+-
  Cast To Single : DataTypeConversion  OutDataTypeStr=single  SaturateOnIntegerOverflow=off  RndMeth=Floor
  Cast To Single1 : DataTypeConversion  OutDataTypeStr=single  SaturateOnIntegerOverflow=off  RndMeth=Floor
  Cast To Single3 : DataTypeConversion  OutDataTypeStr=single  SaturateOnIntegerOverflow=off  RndMeth=Floor
  Constant : Constant  Commented=on  Value=single(0.2)
  Constant1 : Constant  Commented=on  Value=single(10)
  Constant10 : Constant  Value=single(10)
  Constant2 : Constant  Value=single(7/7)
  Constant3 : Constant  Value=boolean(1)
  Constant4 : Constant  Value=boolean(0)
  Constant5 : Constant  Value=boolean(1)
  Constant6 : Constant  Value=single(300)
  Constant7 : Constant  Value=single(0)
  Constant8 : Constant  Commented=on  Value=CurrentBypassValue
  Constant9 : Constant  Value=single(0.2)
  Gain : Gain  Gain=-1
  Gain1 : Gain  Gain=single(7)
  Gain2 : Gain  Commented=on  Gain=1/100
  Gain3 : Gain  Commented=on  Gain=1/100
  Gain4 : Gain  Gain=1/300
  Gain5 : Gain  Gain=1/300
  PI : PID_Lib/PI  SystemSampleTime=-1  VariantActivationTime=update diagram  Latency=0  AutoFrameSizeCalculation=off
  Product : Product
  Scope : Scope
  Step : Step  Time=30  Before=-0.5  After=-1.5
  Step1 : Step  Time=50  Before=200  After=300
  Subsystem5 : Subsystem  Commented=through
  Switch : Switch  Criteria=u2 ~= 0  SaturateOnIntegerOverflow=off  InputSameDT=off
  Terminator{,1..5} (6 alike) : Terminator
  PI_f32DGridCurrentReference : Outport
  MPCC_f32DCLinkFiltered : Outport  Port=2
  MPCC_f32DCLinkref : Outport  Port=3
  wires:
  Add/1 -> PI/1
  Constant2/1 -> Gain/1, PI/4
  Gain/1 -> PI/5
  Constant3/1 -> PI/6
  Constant4/1 -> PI/7
  PI/2 -> Terminator/1
  PI/3 -> Terminator1/1
  PI/4 -> Terminator2/1
  PI/5 -> Terminator3/1
  Constant5/1 -> Switch/2
  PI/1 -> Switch/1, Scope/1
  Switch/1 -> Cast To Single/1
  Cast To Single1/1 -> Gain5/1
  Cast To Single/1 -> Gain1/1
  Cast To Single3/1 -> Gain4/1, MPCC_f32DCLinkref/1
  PI_f32DCLinkVoltage/1 -> Cast To Single1/1, MPCC_f32DCLinkFiltered/1
  Constant7/1 -> PI/8
  Step/1 -> Switch/3
  Gain1/1 -> PI_f32DGridCurrentReference/1
  PI_f32DCLinkVoltageRef/1 -> Terminator4/1
  PI_f32DCLink/1 -> Terminator5/1
  Constant9/1 -> PI/2
  Constant10/1 -> PI/3
  Gain4/1 -> Add/1
  Gain5/1 -> Add/2
  Constant6/1 -> Cast To Single3/1

== system Final_Tune_of_Bandwidth_PI_Result/Subsystem1/ABCtoDQO ==
  PI_f32GridCurrentA : Inport
  PI_f32GridCurrentB : Inport  Port=2
  PI_f32GridCurrentC : Inport  Port=3
  PI_f32GridVoltageA : Inport  Port=4
  PI_f32GridVoltageB : Inport  Port=5
  PI_f32GridVoltageC : Inport  Port=6
  PI_f32ElectricalAngle : Inport  Port=7
  ABCtoDQOCurrent : Subsystem  Commented=on
  ABCtoDQOVoltage : Subsystem  Commented=on
  Ground : Ground
  abc_dq : Subsystem
  abc_dq1 : Subsystem
  PI_f32DGridCurrent : Outport
  PI_f32QGridCurrent : Outport  Port=2
  PI_f32OGridCurrent : Outport  Port=3
  PI_f32DGridVoltage : Outport  Port=4
  PI_f32QGridVoltage : Outport  Port=5
  PI_f32OGridVoltage : Outport  Port=6
  wires:
  abc_dq/1(Id) -> PI_f32DGridCurrent/1
  abc_dq/2(Iq) -> PI_f32QGridCurrent/1
  PI_f32ElectricalAngle/1 -> [PI_f32ElectricalAngle]
  [PI_f32ElectricalAngle] -> abc_dq/1(theta)
  Ground/1 -> PI_f32OGridCurrent/1, PI_f32OGridVoltage/1
  abc_dq1/2(Iq) -> PI_f32QGridVoltage/1
  [PI_f32ElectricalAngle] -> abc_dq1/1(theta)
  abc_dq1/1(Id) -> PI_f32DGridVoltage/1
  PI_f32GridCurrentC/1 -> abc_dq/4(c)
  PI_f32GridCurrentB/1 -> abc_dq/3(b)
  PI_f32GridCurrentA/1 -> abc_dq/2(a)
  PI_f32GridVoltageA/1 -> abc_dq1/2(a)
  PI_f32GridVoltageB/1 -> abc_dq1/3(b)
  PI_f32GridVoltageC/1 -> abc_dq1/4(c)

== system Final_Tune_of_Bandwidth_PI_Result/Subsystem1/CodeGeneration ==
  Input : Inport
  Add : Sum  Inputs=+-  OutDataTypeStr=Inherit: Same as first input
  Demux2 : Demux  Outputs=2
  Index Vector : MultiPortSwitch  Inputs=1  SaturateOnIntegerOverflow=off  InputSameDT=off
  SCI Transmit : c280xlib/SCI Transmit  sciModule=A  dataHead=''  dataTail=''  blockingMode=on  outputStatus=off
  While Iterator : WhileIterator  MaxIters=-1  WhileBlockType=do-while  ShowIterationPort=on  OutputDataType=int16
  wires:
  While Iterator/1 -> Add/2, Index Vector/1
  Demux2/1 -> Index Vector/2
  Index Vector/1 -> SCI Transmit/1
  Add/1 -> While Iterator/1
  Demux2/2 -> Add/1
  Input/1 -> Demux2/1

== system Final_Tune_of_Bandwidth_PI_Result/Subsystem1/Data ==
  Data : Inport
  Data_width : Inport  Port=2
  Action Port : ActionPort  ActionPortLabel=else
  Mux : Mux  Inputs=2
  Start : Constant  Value=hex2dec('0000')  OutDataTypeStr=uint16
  Data_out : Outport  VectorParamsAs1DForOutWhenUnconnected=off
  Iteration : Outport  Port=2  VectorParamsAs1DForOutWhenUnconnected=off
  wires:
  Start/1 -> Mux/2
  Mux/1 -> Data_out/1
  Data/1 -> Mux/1
  Data_width/1 -> Iteration/1

== system Final_Tune_of_Bandwidth_PI_Result/Subsystem1/Data_Conditioning ==
  In1 : Inport
  Data Type Conversion3 : DataTypeConversion  OutDataTypeStr=uint16  ConvertRealWorld=Stored Integer (SI)  SaturateOnIntegerOverflow=off  RndMeth=Floor
  Out1 : Outport  VectorParamsAs1DForOutWhenUnconnected=off
  wires:
  Data Type Conversion3/1 -> Out1/1
  In1/1 -> Data Type Conversion3/1

== system Final_Tune_of_Bandwidth_PI_Result/Subsystem1/Decoupling_Loop ==
  PI_f32DGridCurrent : Inport
  PI_f32QGridCurrent : Inport  Port=2
  PI_f32DGridVoltage : Inport  Port=3
  PI_f32QGridVoltage : Inport  Port=4
  PI_f32AngularFrequency : Inport  Port=5
  PI_f32DCLinkVoltage : Inport  Port=6
  PI_f32LGrid : Inport  Port=7
  PI_f32DVoltage : Inport  Port=8
  PI_f32QVoltage : Inport  Port=9
  PI_f32ElectricalAngle : Inport  Port=10
  ABCtoDQOVoltage : Subsystem  Commented=on
  Cast To Single : DataTypeConversion  OutDataTypeStr=single  SaturateOnIntegerOverflow=off  RndMeth=Floor
  Cast To Single1 : DataTypeConversion  OutDataTypeStr=single  SaturateOnIntegerOverflow=off  RndMeth=Floor
  Cast To Single2 : DataTypeConversion  OutDataTypeStr=single  SaturateOnIntegerOverflow=off  RndMeth=Floor
  Constant : Constant  Value=single(0)
  Decoupling_Loop : Subsystem
  Saturation : Saturate  Commented=on  UpperLimit=single(2/sqrt(3))  LowerLimit=single(-2/sqrt(3))
  Saturation1 : Saturate  Commented=on  UpperLimit=single(2/sqrt(3))  LowerLimit=single(-2/sqrt(3))
  Scope : Scope
  Scope1 : Scope
  Terminator : Terminator
  dq_abc : Subsystem
  PI_f32MAVoltageRef : Outport
  PI_f32MBVoltageRef : Outport  Port=2
  PI_f32MCVoltageRef : Outport  Port=3
  wires:
  PI_f32DGridCurrent/1 -> Decoupling_Loop/1(PI_f32DGridCurrent)
  PI_f32QGridCurrent/1 -> Decoupling_Loop/2(PI_f32QGridCurrent)
  PI_f32DGridVoltage/1 -> Decoupling_Loop/3(PI_f32DGridVoltage)
  PI_f32QGridVoltage/1 -> Decoupling_Loop/4(PI_f32QGridVoltage)
  PI_f32AngularFrequency/1 -> Decoupling_Loop/5(PI_f32AngularFrequency)
  PI_f32LGrid/1 -> Decoupling_Loop/7(PI_f32LGrid)
  PI_f32DVoltage/1 -> Decoupling_Loop/8(PI_f32DVoltage)
  PI_f32QVoltage/1 -> Decoupling_Loop/9(PI_f32QVoltage)
  PI_f32ElectricalAngle/1 -> [PI_f32ElectricalAngle]
  PI_f32DCLinkVoltage/1 -> Decoupling_Loop/6(PI_f32DCLinkVoltage)
  [PI_f32ElectricalAngle] -> dq_abc/1(theta)
  Constant/1 -> Terminator/1
  [PI_f32MDVoltageRef] -> dq_abc/2(vd)
  [PI_f32MQVoltageRef] -> dq_abc/3(vq)
  dq_abc/2(Ib) -> Cast To Single1/1
  dq_abc/3(Ic) -> Cast To Single2/1
  dq_abc/1(Ia) -> Cast To Single/1
  Decoupling_Loop/1(PI_f32MDVoltageRef) -> [PI_f32MDVoltageRef]
  Decoupling_Loop/2(PI_f32MQVoltageRef) -> [PI_f32MQVoltageRef]
  Cast To Single/1 -> PI_f32MAVoltageRef/1
  Cast To Single1/1 -> PI_f32MBVoltageRef/1
  Cast To Single2/1 -> PI_f32MCVoltageRef/1

== system Final_Tune_of_Bandwidth_PI_Result/Subsystem1/End ==
  Data : Inport
  Data_width : Inport  Port=2
  Action Port : ActionPort  ActionPortLabel=elseif(u1 == 599)
  Bias : Bias  Bias=1  SaturateOnIntegerOverflow=off
  Mux : Mux  Inputs=2
  Start : Constant  Value=hex2dec('4545')  OutDataTypeStr=uint16
  Data_out : Outport  VectorParamsAs1DForOutWhenUnconnected=off
  Iteration : Outport  Port=2  VectorParamsAs1DForOutWhenUnconnected=off
  wires:
  Mux/1 -> Data_out/1
  Data_width/1 -> Bias/1
  Start/1 -> Mux/2
  Bias/1 -> Iteration/1
  Data/1 -> Mux/1

== system Final_Tune_of_Bandwidth_PI_Result/Subsystem1/IIR ==
  IIR_IN : Inport
  Add : Sum
  Constant : Constant
  Constant1 : Constant  Value=0.1
  Gain : Gain  Gain=0.1
  Product : Product
  Subtract : Sum  Inputs=+-
  Unit Delay : UnitDelay  SampleTime=-1  HasFrameUpgradeWarning=on
  IIR_OUT : Outport
  wires:
  Add/1 -> IIR_OUT/1, Unit Delay/1
  Gain/1 -> Add/1
  Unit Delay/1 -> Product/2
  Subtract/1 -> Product/1
  Product/1 -> Add/2
  IIR_IN/1 -> Gain/1
  Constant/1 -> Subtract/1
  Constant1/1 -> Subtract/2

== system Final_Tune_of_Bandwidth_PI_Result/Subsystem1/LPF1 ==
  u_k : Inport
  Add : Sum  Inputs=+-
  Add1 : Sum
  Delay : Delay  DelayLength=1
  Gain : Gain  Gain=single(100/600)
  y_k : Outport
  wires:
  Delay/1 -> Add/2, Add1/2
  Add/1 -> Gain/1
  Gain/1 -> Add1/1
  Add1/1 -> y_k/1, Delay/1
  u_k/1 -> Add/1

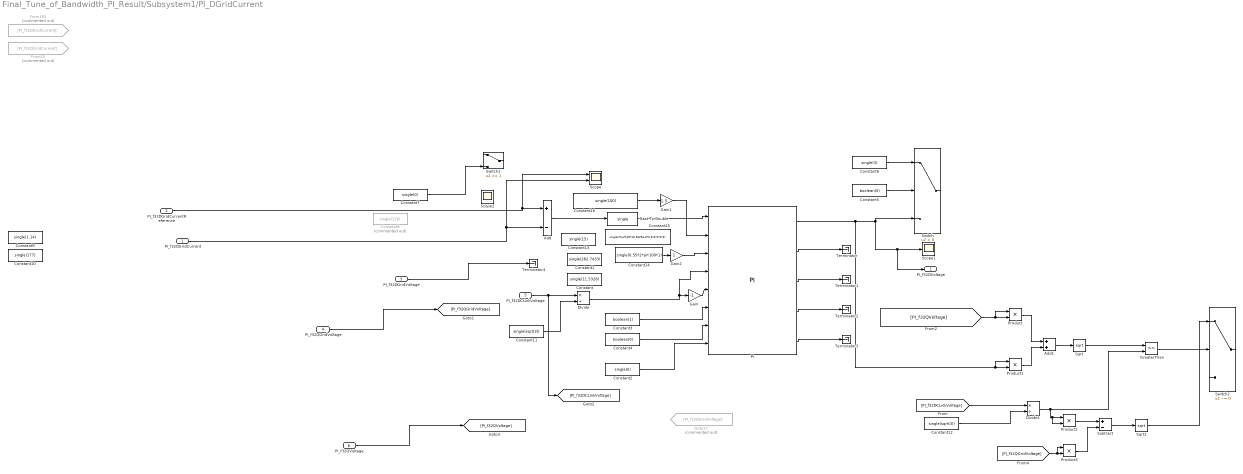
== system Final_Tune_of_Bandwidth_PI_Result/Subsystem1/PI_DGridCurrent ==
  PI_f32DGridCurrent : Inport
  PI_f32DGridCurrentReference : Inport  Port=2
  PI_f32DGridVoltage : Inport  Port=3
  PI_f32QGridVoltage : Inport  Port=4
  PI_f32DCLinkVoltage : Inport  Port=5
  PI_f32QVoltage : Inport  Port=6
  Add : Sum  Inputs=+-
  Add1 : Sum
  Cast To Double : DataTypeConversion  OutDataTypeStr=single  SaturateOnIntegerOverflow=off  RndMeth=Floor
  Constant : Constant  Value=single(11.5328)
  Constant1 : Constant  Value=single(282.7433)
  Constant10 : Constant  Value=single(177)
  Constant11 : Constant  Value=single(sqrt(3))
  Constant12 : Constant  Value=single(sqrt(3))
  Constant13 : Constant  Value=single(15)
  Constant14 : Constant  Value=single(0.55*2*pi*100*1)
  Constant15 : Constant  Value=single(2*pi*100*18.5825e-3*0.3*2*2*2*3)
  Constant16 : Constant  Value=single(100)
  Constant2 : Constant  Value=single(0)
  Constant3 : Constant  Value=boolean(1)
  Constant4 : Constant  Value=boolean(0)
  Constant5 : Constant  Value=boolean(0)
  Constant6 : Constant  Value=single(3)
  Constant7 : Constant  Value=single(0)
  Constant8 : Constant  Commented=on  Value=single(156)
  Constant9 : Constant  Value=single(1.14)
  Divide : Product  Inputs=*/  RndMeth=Zero  SaturateOnIntegerOverflow=on
  Divide1 : Product  Inputs=*/  RndMeth=Zero  SaturateOnIntegerOverflow=on
  From15 : From  Commented=on  GotoTag=PI_f32QGridCurrent
  From153 : From  Commented=on  GotoTag=PI_f32DGridCurrent
  Gain : Gain  Gain=-1
  Gain1 : Gain  Gain=1.5
  Gain2 : Gain
  Goto27 : Goto  Commented=on  GotoTag=PI_f32DGridVoltage
  GreaterThan : RelationalOperator  OutDataTypeStr=boolean  RndMeth=Simplest  InputSameDT=off
  PI : PID_Lib/PI  SystemSampleTime=-1  VariantActivationTime=update diagram  Latency=0  AutoFrameSizeCalculation=off
  Product{,1..3} (4 alike) : Product
  Scope : Scope  NumInputPorts=2
  Scope1 : Scope
  Scope2 : Scope
  Sqrt : Sqrt
  Sqrt1 : Sqrt
  Subtract : Sum  Inputs=+-
  Switch : Switch  Criteria=u2 > Threshold  SaturateOnIntegerOverflow=off  InputSameDT=off
  Switch1 : Switch  Threshold=1  SaturateOnIntegerOverflow=off  InputSameDT=off
  Switch2 : Switch  Criteria=u2 ~= 0  SaturateOnIntegerOverflow=off  InputSameDT=off
  Terminator{,1..4} (5 alike) : Terminator
  PI_f32DVoltage : Outport
  wires:
  PI_f32DGridCurrent/1 -> Scope/2, Add/2
  Gain/1 -> PI/5
  Constant3/1 -> PI/6
  Constant4/1 -> PI/7
  PI/2 -> Terminator/1
  PI/3 -> Terminator1/1
  PI/4 -> Terminator2/1
  PI/5 -> Terminator3/1
  Constant5/1 -> Switch/2
  Constant6/1 -> Switch/1
  Cast To Double/1 -> PI/1
  Add/1 -> Cast To Double/1
  Constant7/1 -> Switch1/3
  PI_f32DGridCurrentReference/1 -> Scope/1, Add/1
  Constant2/1 -> PI/8
  PI_f32DGridVoltage/1 -> Terminator4/1
  PI_f32QGridVoltage/1 -> [PI_f32QGridVoltage]
  Add1/1 -> Sqrt/1
  Product1/1 -> Add1/2
  Product/1 -> Add1/1
  [PI_f32QVoltage] -> Product/1, Product/2
  PI/1 -> Product1/1, Product1/2, Switch/3, PI_f32DVoltage/1, Scope1/1
  PI_f32DCLinkVoltage/1 -> [PI_f32DCLinkVoltage], Divide/1
  Constant11/1 -> Divide/2
  Constant12/1 -> Divide1/2
  [PI_f32DCLinkVoltage] -> Divide1/1
  Sqrt/1 -> GreaterThan/1
  Divide1/1 -> Product2/2, Product2/1, GreaterThan/2
  GreaterThan/1 -> Switch2/2
  Product2/1 -> Subtract/1
  [PI_f32QGridVoltage] -> Product3/1, Product3/2
  Product3/1 -> Subtract/2
  Subtract/1 -> Sqrt1/1
  Sqrt1/1 -> Switch2/1
  Divide/1 -> PI/4, Gain/1
  PI_f32QVoltage/1 -> [PI_f32QVoltage]
  Constant14/1 -> Gain2/1
  Constant16/1 -> Gain1/1
  Gain1/1 -> PI/2
  Gain2/1 -> PI/3

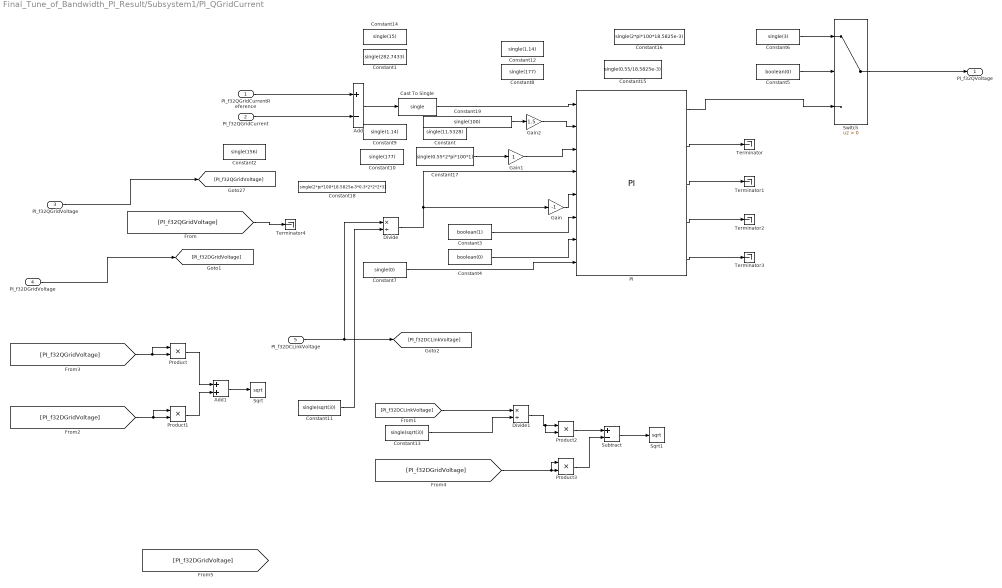
== system Final_Tune_of_Bandwidth_PI_Result/Subsystem1/PI_QGridCurrent ==
  PI_f32QGridCurrentReference : Inport
  PI_f32QGridCurrent : Inport  Port=2
  PI_f32QGridVoltage : Inport  Port=3
  PI_f32DGridVoltage : Inport  Port=4
  PI_f32DCLinkVoltage : Inport  Port=5
  Add : Sum  Inputs=+-
  Add1 : Sum
  Cast To Single : DataTypeConversion  OutDataTypeStr=single  SaturateOnIntegerOverflow=off  RndMeth=Floor
  Constant : Constant  Value=single(11.5328)
  Constant1 : Constant  Value=single(282.7433)
  Constant10 : Constant  Value=single(177)
  Constant11 : Constant  Value=single(sqrt(3))
  Constant12 : Constant  Value=single(1.14)
  Constant13 : Constant  Value=single(sqrt(3))
  Constant14 : Constant  Value=single(15)
  Constant15 : Constant  Value=single(0.55/18.5825e-3)
  Constant16 : Constant  Value=single(2*pi*100*18.5825e-3)
  Constant17 : Constant  Value=single(0.55*2*pi*100*1)
  Constant18 : Constant  Value=single(2*pi*100*18.5825e-3*0.3*2*2*2*3)
  Constant19 : Constant  Value=single(100)
  Constant2 : Constant  Value=single(156)
  Constant3 : Constant  Value=boolean(1)
  Constant4 : Constant  Value=boolean(0)
  Constant5 : Constant  Value=boolean(0)
  Constant6 : Constant  Value=single(3)
  Constant7 : Constant  Value=single(0)
  Constant8 : Constant  Value=single(177)
  Constant9 : Constant  Value=single(1.14)
  Divide : Product  Inputs=*/  RndMeth=Zero  SaturateOnIntegerOverflow=on
  Divide1 : Product  Inputs=*/  RndMeth=Zero  SaturateOnIntegerOverflow=on
  Gain : Gain  Gain=-1
  Gain1 : Gain
  Gain2 : Gain  Gain=1.5
  PI : PID_Lib/PI  SystemSampleTime=-1  VariantActivationTime=update diagram  Latency=0  AutoFrameSizeCalculation=off
  Product{,1..3} (4 alike) : Product
  Sqrt : Sqrt
  Sqrt1 : Sqrt
  Subtract : Sum  Inputs=+-
  Switch : Switch  Criteria=u2 > Threshold  SaturateOnIntegerOverflow=off  InputSameDT=off
  Terminator{,1..4} (5 alike) : Terminator
  PI_f32QVoltage : Outport
  wires:
  PI_f32QGridCurrentReference/1 -> Add/1
  PI_f32QGridCurrent/1 -> Add/2
  Add/1 -> Cast To Single/1
  Gain/1 -> PI/5
  Constant3/1 -> PI/6
  Constant4/1 -> PI/7
  PI/2 -> Terminator/1
  PI/3 -> Terminator1/1
  PI/4 -> Terminator2/1
  PI/5 -> Terminator3/1
  Constant5/1 -> Switch/2
  Constant6/1 -> Switch/1
  Switch/1 -> PI_f32QVoltage/1
  Cast To Single/1 -> PI/1
  PI/1 -> Switch/3
  Constant7/1 -> PI/8
  PI_f32QGridVoltage/1 -> [PI_f32QGridVoltage]
  [PI_f32QGridVoltage] -> Terminator4/1
  PI_f32DGridVoltage/1 -> [PI_f32DGridVoltage]
  Product/1 -> Add1/1
  [PI_f32DGridVoltage] -> Product1/1, Product1/2
  [PI_f32QGridVoltage] -> Product/1, Product/2
  Product1/1 -> Add1/2
  Add1/1 -> Sqrt/1
  Constant11/1 -> Divide/2
  Subtract/1 -> Sqrt1/1
  [PI_f32DCLinkVoltage] -> Divide1/1
  [PI_f32DGridVoltage] -> Product3/1, Product3/2
  Product3/1 -> Subtract/2
  Product2/1 -> Subtract/1
  Divide1/1 -> Product2/2, Product2/1
  Constant13/1 -> Divide1/2
  PI_f32DCLinkVoltage/1 -> Divide/1, [PI_f32DCLinkVoltage]
  Divide/1 -> Gain/1, PI/4
  Constant17/1 -> Gain1/1
  Constant19/1 -> Gain2/1
  Gain1/1 -> PI/3
  Gain2/1 -> PI/2
